simulink model "thermostat_exec"  (Simulink 3.00)
libraries: execlib x6

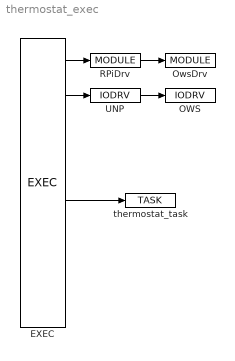
== system thermostat_exec ==
  EXEC : execlib/EXEC  target=PC - Linux  tick=1  ntick0=1  ntick1=4  ntick2=4  ntick3=1200  pri0=5  pri1=9  pri2=13  pri3=18
  OWS : execlib/IODRV  module=OwsDrv  classname=OwsDrv  cfgname=thermostat_owscfg.rio  factor=1  stack=10240  pri=3  timer=off
  OwsDrv : execlib/MODULE
  RPiDrv : execlib/MODULE
  UNP : execlib/IODRV  module=RPiDrv  classname=UnpDrv  factor=1  stack=10240  pri=3  timer=off
  thermostat_task : execlib/TASK  factor=1  start=0  stop=1  stack=10240  MDLOPEN=on
  wires:
  EXEC/1 -> RPiDrv/1
  EXEC/2 -> UNP/1
  EXEC/5 -> thermostat_task/1
  RPiDrv/1 -> OwsDrv/1
  UNP/1 -> OWS/1
